simulink model "gru_quadcl"  (Simulink 8.3)
settings: Solver=FixedStepDiscrete  SolverMode=SingleTasking  StartTime=0.0  StopTime=10  FixedStep=0.01  RelTol=1e-3
undefined symbols (not defined in the file): DiscIntNeverNeededParam
libraries: controllibrary x11, simulink x8, snap2lib x3, simulink_need_slupdate x3, utilitylib x2
settings Model: Creator=simon  LastModifiedBy=Robin
settings DataIOCC: LimitDataPoints=off  SaveOutput=off  SignalLogging=off  SaveTime=off
settings OptimizationCC: InlineParams=on  InlineInvariantSignals=on  ExpressionDepthLimit=2147483647  InitFltsAndDblsToZero=on  OptimizeModelRefInitCode=on  LifeSpan=1
settings DebuggingCC: SaveWithParameterizedLinksMsg=none  SignalResolutionControl=TryResolveAllWithWarning  MultiTaskDSMMsg=warning  MultiTaskCondExecSysMsg=none  FcnCallInpInsideContextMsg=UseLocalSettings
settings HardwareCC: TargetLongLongMode=on  TargetIntDivRoundTo=Zero  TargetEndianess=LittleEndian  TargetHWDeviceType=MATLAB Host  ProdEqTarget=off
settings ModelReferenceCC: ModelReferenceNumInstancesAllowed=Single
settings SFSimCC: SimParseCustomCode=off
settings RTWCC: SystemTargetFile=ert_shrlib.tlc  GenCodeOnly=on  TemplateMakefile=ert_default_tmf  PostCodeGenCommand=packNGo(buildInfo, {'packType' 'hierarchical'})  Description=Embedded Coder (host-based shared library target)  ProcessScript=ert_shrlib_make_rtw_hook  IncludeERTFirstTime=on
settings CodeAppCC: IgnoreCustomStorageClasses=off
settings STFCustomTargetCC: GenerateSampleERTMain=on  ParMdlRefBuildCompliant=on  CompOptLevelCompliant=on  CombineOutputUpdateFcns=on  ERTCustomFileBanners=on  SupportContinuousTime=off  SupportNonInlinedSFcns=off  MATLABClassNameForMDSCustomization=Simulink.SoftwareTarget.ERTCustomization  ModelStepFunctionPrototypeControlCompliant=on  GRTInterface=off  SystemTargetFile=ert_shrlib.tlc
settings ERTTargetCC: MultiwordLength=2048  GenerateSampleERTMain=on  ConcurrentExecutionCompliant=off  ERTFirstTimeCompliant=off  CPPClassGenCompliant=off  InlinedParameterPlacement=NonHierarchical  ERTCustomFileTemplate=example_file_process.tlc  ConvertIfToSwitch=off  SuppressUnreachableDefaultCases=off

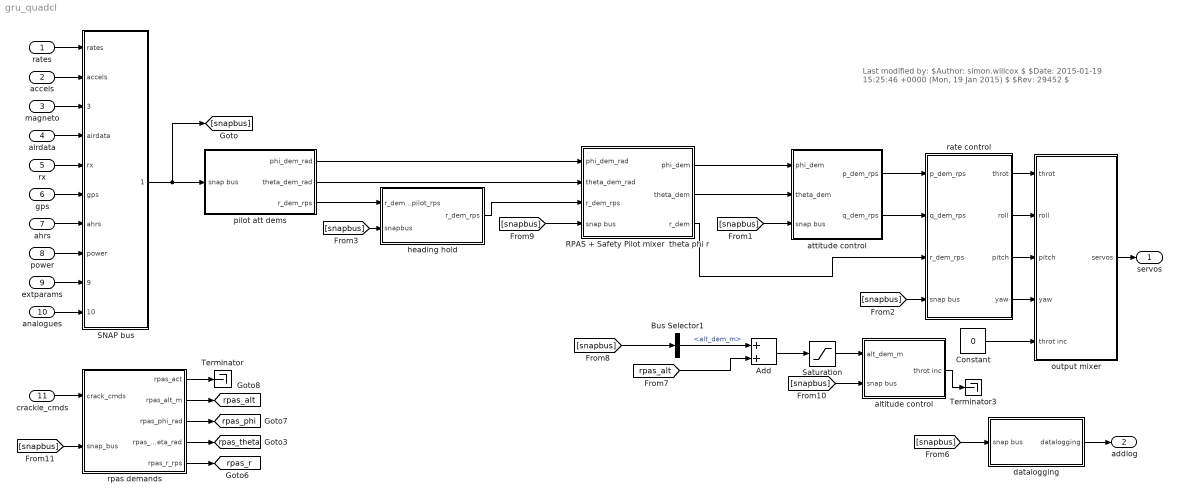
== system gru_quadcl ==
  note: Last modified by:
      | $Author: simon.willcox $
      | $Date: 2015-01-19 15:25:46 +0000 (Mon, 19 Jan 2015) $
      | $Rev: 29452 $
  rates : Inport  PortDimensions=3  SampleTime=0.01
  accels : Inport  Port=2  PortDimensions=3  SampleTime=0.01
  magneto : Inport  Port=3  PortDimensions=3  SampleTime=0.01
  airdata : Inport  Port=4  PortDimensions=3  SampleTime=0.01
  rx : Inport  Port=5  PortDimensions=8  SampleTime=0.01
  gps : Inport  Port=6  PortDimensions=9  SampleTime=0.01
  ahrs : Inport  Port=7  PortDimensions=4  SampleTime=0.01
  power : Inport  Port=8  PortDimensions=3  SampleTime=0.01
  extparams : Inport  Port=9  PortDimensions=64  SampleTime=0.01
  analogues : Inport  Port=10  PortDimensions=8  SampleTime=0.01
  crackle_cmds : Inport  Port=11  PortDimensions=32  SampleTime=0.01
  Add : Sum
  Bus Selector1 : BusSelector  OutputSignals=extbus.alt_dem_m
  Constant : Constant  Value=0
  RPAS + Safety Pilot mixer  theta phi r : Subsystem
  SNAP bus : Subsystem
  Saturation : Saturate  UpperLimit=5  LowerLimit=0
  Terminator : Terminator
  Terminator3 : Terminator
  altitude control : Subsystem
  attitude control : Subsystem
  datalogging : Subsystem  AncestorBlock=snap2lib/datalogging
  heading hold : Subsystem
  output mixer : Subsystem
  pilot att dems : Subsystem
  rate control : Subsystem
  rpas demands : Subsystem
  servos : Outport  PortDimensions=8
  addlog : Outport  Port=2  PortDimensions=32
  tag scope: rpas_alt=global, rpas_phi=global, rpas_r=global, rpas_theta=global
  wires:
  rates/1 -> SNAP bus/1(rates)
  accels/1 -> SNAP bus/2(accels)
  airdata/1 -> SNAP bus/4(airdata)
  power/1 -> SNAP bus/8(power)
  rx/1 -> SNAP bus/5(rx)
  gps/1 -> SNAP bus/6(gps)
  datalogging/1(datalogging) -> addlog/1
  ahrs/1 -> SNAP bus/7(ahrs)
  extparams/1 -> SNAP bus/9(extparams)
  output mixer/1(servos) -> servos/1
  magneto/1 -> SNAP bus/3(magneto)
  analogues/1 -> SNAP bus/10(analogues)
  rate control/1(throt) -> output mixer/1(throt)
  rate control/2(roll) -> output mixer/2(roll)
  [snapbus] -> datalogging/1(snap bus)
  rate control/4(yaw) -> output mixer/4(yaw)
  rate control/3(pitch) -> output mixer/3(pitch)
  SNAP bus/1(snap bus) -> [snapbus], pilot att dems/1(snap bus)
  [snapbus] -> attitude control/3(snap bus)
  [snapbus] -> rate control/4(snap bus)
  Saturation/1 -> altitude control/1(alt_dem_m)
  [snapbus] -> Bus Selector1/1
  rpas demands/1(rpas_act) -> Terminator/1
  rpas demands/2(rpas_alt_m) -> [rpas_alt]
  rpas demands/5(rpas_r_rps) -> [rpas_r]
  rpas demands/3(rpas_phi_rad) -> [rpas_phi]
  rpas demands/4(rpas_theta_rad) -> [rpas_theta]
  [snapbus] -> rpas demands/2(snap_bus)
  crackle_cmds/1 -> rpas demands/1(crack_cmds)
  pilot att dems/1(phi_dem_rad) -> RPAS + Safety Pilot mixer  theta phi r/1(phi_dem_rad)
  RPAS + Safety Pilot mixer  theta phi r/1(phi_dem) -> attitude control/1(phi_dem)
  pilot att dems/2(theta_dem_rad) -> RPAS + Safety Pilot mixer  theta phi r/2(theta_dem_rad)
  RPAS + Safety Pilot mixer  theta phi r/2(theta_dem) -> attitude control/2(theta_dem)
  RPAS + Safety Pilot mixer  theta phi r/3(r_dem) -> rate control/3(r_dem_rps)
  [snapbus] -> RPAS + Safety Pilot mixer  theta phi r/4(snap bus)
  Bus Selector1/1 -> Add/1  "<alt_dem_m>"
  [rpas_alt] -> Add/2
  Add/1 -> Saturation/1
  [snapbus] -> altitude control/2(snap bus)
  altitude control/1(throt inc) -> Terminator3/1
  attitude control/1(p_dem_rps) -> rate control/1(p_dem_rps)
  attitude control/2(q_dem_rps) -> rate control/2(q_dem_rps)
  Constant/1 -> output mixer/5(throt inc)
  [snapbus] -> heading hold/2(snapbus)
  pilot att dems/3(r_dem_rps) -> heading hold/1(r_dem_pilot_rps)
  heading hold/1(r_dem_rps) -> RPAS + Safety Pilot mixer  theta phi r/3(r_dem_rps)

== system gru_quadcl/RPAS + Safety Pilot mixer  theta phi r ==
  phi_dem_rad : Inport
  theta_dem_rad : Inport  Port=2
  r_dem_rps : Inport  Port=3
  snap bus : Inport  Port=4
  Add : Sum
  Add1 : Sum
  Bus Selector5 : BusSelector  OutputSignals=rx.snapact
  Switch3 : Switch  Threshold=0.5
  Switch4 : Switch  Threshold=0.5
  phi_dem : Outport
  theta_dem : Outport  Port=2
  r_dem : Outport  Port=3
  wires:
  phi_dem_rad/1 -> Switch4/3, Add/2
  theta_dem_rad/1 -> Switch3/3, Add1/2
  Add/1 -> Switch4/1
  Add1/1 -> Switch3/1
  Switch4/1 -> phi_dem/1
  Switch3/1 -> theta_dem/1
  r_dem_rps/1 -> r_dem/1
  [rpas_phi] -> Add/1
  [rpas_theta] -> Add1/1
  snap bus/1 -> Bus Selector5/1
  Bus Selector5/1 -> Switch3/2, Switch4/2  "<snapact>"

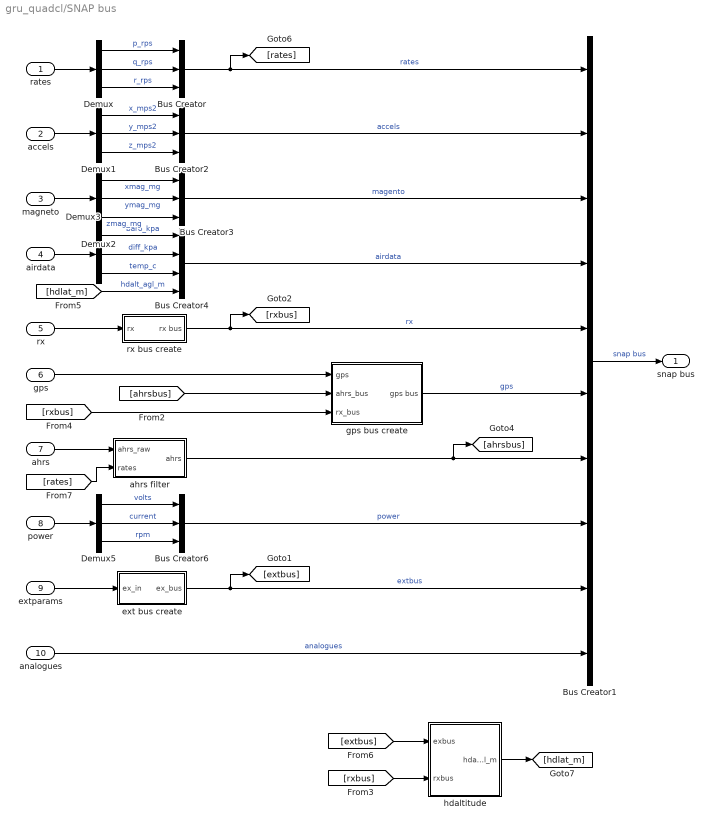
== system gru_quadcl/SNAP bus ==
  rates : Inport  PortDimensions=3
  accels : Inport  Port=2  PortDimensions=3
  magneto : Inport  Port=3  PortDimensions=3
  airdata : Inport  Port=4  PortDimensions=3
  rx : Inport  Port=5  PortDimensions=8
  gps : Inport  Port=6  PortDimensions=9
  ahrs : Inport  Port=7  PortDimensions=4
  power : Inport  Port=8  PortDimensions=3
  extparams : Inport  Port=9  PortDimensions=64
  analogues : Inport  Port=10  PortDimensions=8
  Bus Creator{,2..3,6} (4 alike) : BusCreator  Inputs=3
  Bus Creator1 : BusCreator  Inputs=10
  Bus Creator4 : BusCreator
  Demux{,1..3,5} (5 alike) : Demux  Outputs=3
  ahrs filter : Subsystem
  ext bus create : Subsystem
  gps bus create : Subsystem
  hdaltitude : Subsystem
  rx bus create : Subsystem
  snap bus : Outport
  wires:
  Bus Creator1/1 -> snap bus/1  "snap bus"
  Bus Creator6/1 -> Bus Creator1/8  "power"
  power/1 -> Demux5/1
  Demux5/1 -> Bus Creator6/1  "volts"
  Demux5/2 -> Bus Creator6/2  "current"
  Demux5/3 -> Bus Creator6/3  "rpm"
  ahrs filter/1(ahrs) -> Bus Creator1/7, [ahrsbus]
  ahrs/1 -> ahrs filter/1(ahrs_raw)
  gps bus create/1(gps bus) -> Bus Creator1/6  "gps"
  gps/1 -> gps bus create/1(gps)
  rx bus create/1(rx bus) -> Bus Creator1/5, [rxbus]  "rx"
  Bus Creator4/1 -> Bus Creator1/4  "airdata"
  airdata/1 -> Demux3/1
  Demux3/1 -> Bus Creator4/1  "baro_kpa"
  Demux3/2 -> Bus Creator4/2  "diff_kpa"
  Demux3/3 -> Bus Creator4/3  "temp_c"
  Bus Creator3/1 -> Bus Creator1/3  "magento"
  magneto/1 -> Demux2/1
  Demux2/1 -> Bus Creator3/1  "xmag_mg"
  Demux2/2 -> Bus Creator3/2  "ymag_mg"
  Demux2/3 -> Bus Creator3/3  "zmag_mg"
  Bus Creator2/1 -> Bus Creator1/2  "accels"
  accels/1 -> Demux1/1
  Demux1/1 -> Bus Creator2/1  "x_mps2"
  Demux1/2 -> Bus Creator2/2  "y_mps2"
  Demux1/3 -> Bus Creator2/3  "z_mps2"
  rx/1 -> rx bus create/1(rx)
  rates/1 -> Demux/1
  Bus Creator/1 -> Bus Creator1/1, [rates]  "rates"
  Demux/1 -> Bus Creator/1  "p_rps"
  Demux/2 -> Bus Creator/2  "q_rps"
  Demux/3 -> Bus Creator/3  "r_rps"
  extparams/1 -> ext bus create/1(ex_in)
  ext bus create/1(ex_bus) -> Bus Creator1/9, [extbus]  "extbus"
  analogues/1 -> Bus Creator1/10  "analogues"
  [rxbus] -> gps bus create/3(rx_bus)
  [ahrsbus] -> gps bus create/2(ahrs_bus)
  [rxbus] -> hdaltitude/2(rxbus)
  [extbus] -> hdaltitude/1(exbus)
  [rates] -> ahrs filter/2(rates)
  hdaltitude/1(hdalt_agl_m) -> [hdlat_m]
  [hdlat_m] -> Bus Creator4/4  "hdalt_agl_m"

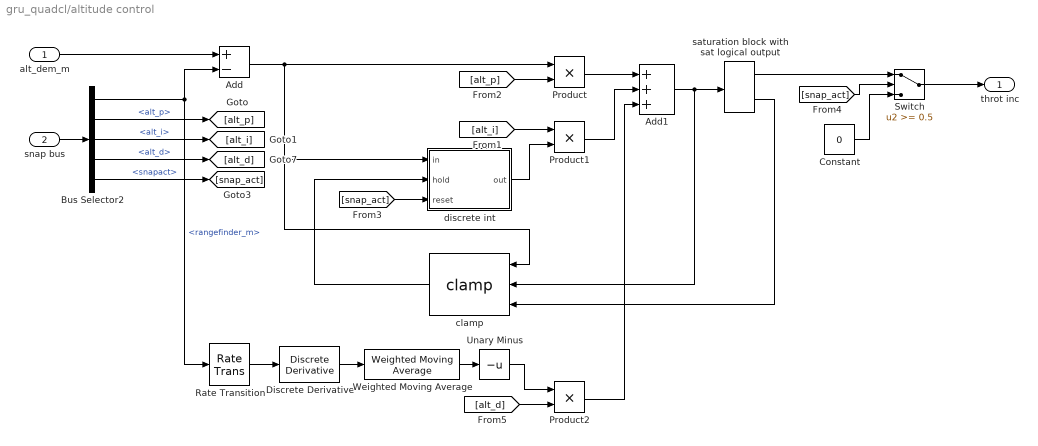
== system gru_quadcl/altitude control ==
  alt_dem_m : Inport
  snap bus : Inport  Port=2
  Add : Sum  Inputs=+-
  Add1 : Sum  Inputs=+++
  Bus Selector2 : BusSelector  OutputSignals=extbus.rangefinder_m,extbus.alt_p,extbus.alt_i,extbus.alt_d,rx.snapact
  Constant : Constant  Value=0
  Discrete Derivative : simulink/Discrete/Discrete Derivative  gainval=1.0  ICPrevScaledInput=0.0  InputProcessing=Inherited  OutMin=[]  OutMax=[]  OutDataType=sfix(16)  OutScaling=2^-10  DoSatur=off
  Product : Product  RndMeth=Zero
  Product1 : Product  RndMeth=Zero
  Product2 : Product  RndMeth=Zero
  Rate Transition : RateTransition  OutPortSampleTime=0.1
  Switch : Switch  Threshold=0.5
  Unary Minus : UnaryMinus
  Weighted Moving Average : simulink_need_slupdate/Weighted Moving Average  mgainval=[0.1 0.1 0.1 0.1 0.1 0.1 0.1 0.1 0.1 0.1]  vinit=0.0  samptime=-1  OutDataType=sfix(16)  OutScaling=2^-10  DoSatur=off  GainDataType=sfix( 16 )  MatRadixGroup=Best Precision: Matrix-wise  GainScaling=2^-10
  clamp : controllibrary/clamp
  discrete int : Subsystem
  saturation block with sat logical output : controllibrary/saturation block with sat logical output  ulim=0.4  llim=-0.25
  throt inc : Outport
  wires:
  [snap_act] -> Switch/2
  Constant/1 -> Switch/3
  Switch/1 -> throt inc/1
  saturation block with sat logical output/1 -> Switch/1
  Bus Selector2/4 -> [alt_d]  "<alt_d>"
  Bus Selector2/5 -> [snap_act]  "<snapact>"
  Bus Selector2/3 -> [alt_i]  "<alt_i>"
  Bus Selector2/2 -> [alt_p]  "<alt_p>"
  saturation block with sat logical output/2 -> clamp/3
  [snap_act] -> discrete int/3(reset)
  [alt_i] -> Product1/1
  [alt_p] -> Product/2
  clamp/1 -> discrete int/2(hold)
  Product1/1 -> Add1/2
  discrete int/1(out) -> Product1/2
  Add1/1 -> clamp/2, saturation block with sat logical output/1
  Product/1 -> Add1/1
  Bus Selector2/1 -> Add/2, Rate Transition/1  "<rangefinder_m>"
  Add/1 -> clamp/1, discrete int/1(in), Product/1
  snap bus/1 -> Bus Selector2/1
  alt_dem_m/1 -> Add/1
  Product2/1 -> Add1/3
  [alt_d] -> Product2/2
  Discrete Derivative/1 -> Weighted Moving Average/1
  Weighted Moving Average/1 -> Unary Minus/1
  Unary Minus/1 -> Product2/1
  Rate Transition/1 -> Discrete Derivative/1

== system gru_quadcl/attitude control ==
  phi_dem : Inport
  theta_dem : Inport  Port=2
  snap bus : Inport  Port=3
  pitch att : Subsystem
  roll att : Subsystem
  snap bus1 : InportShadow  Port=3
  p_dem_rps : Outport
  q_dem_rps : Outport  Port=2
  wires:
  snap bus/1 -> roll att/2(snap bus)
  roll att/1(p_dem_rps) -> p_dem_rps/1
  pitch att/1(q_dem_rps) -> q_dem_rps/1
  snap bus1/1 -> pitch att/2(snap bus)
  phi_dem/1 -> roll att/1(phi_dem_rad)
  theta_dem/1 -> pitch att/1(theta_dem_rad)

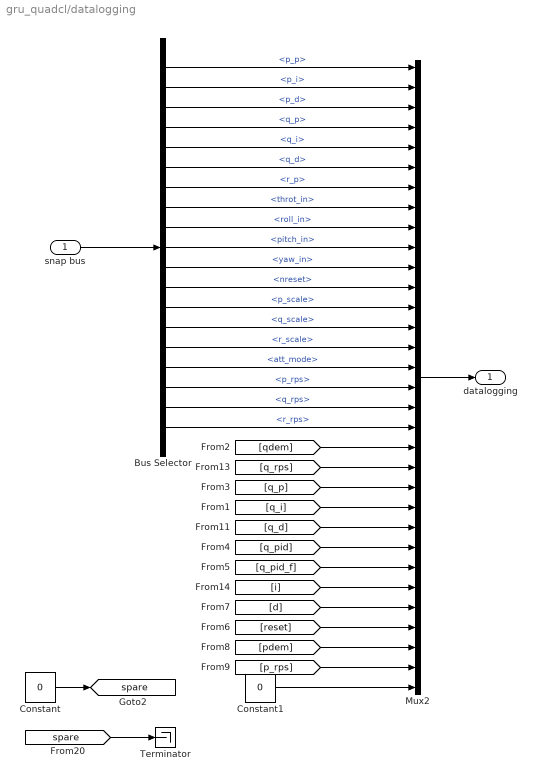
== system gru_quadcl/datalogging ==
  snap bus : Inport
  Bus Selector : BusSelector  OutputSignals=extbus.p_p,extbus.p_i,extbus.p_d,extbus.q_p,extbus.q_i,extbus.q_d,extbus.r_p,rx.throt_in,rx.roll_in,rx.pitch_in,rx.yaw_in,rx.nreset,extbus.p_scale,extbus.q_scale,extbus.r_scale,extbus.att_mode,rates.p_rps,rates.q_rps,rates.r_rps
  Constant : Constant  Value=0
  Constant1 : Constant  Value=0
  Mux2 : Mux  Inputs=32
  Terminator : Terminator
  datalogging : Outport
  tag scope: spare=global
  wires:
  Mux2/1 -> datalogging/1
  Constant/1 -> [spare]
  [spare] -> Terminator/1
  snap bus/1 -> Bus Selector/1
  Bus Selector/1 -> Mux2/1  "<p_p>"
  Bus Selector/3 -> Mux2/3  "<p_d>"
  Bus Selector/2 -> Mux2/2  "<p_i>"
  Bus Selector/7 -> Mux2/7  "<r_p>"
  Bus Selector/8 -> Mux2/8  "<throt_in>"
  Bus Selector/13 -> Mux2/13  "<p_scale>"
  Bus Selector/14 -> Mux2/14  "<q_scale>"
  Bus Selector/11 -> Mux2/11  "<yaw_in>"
  Bus Selector/12 -> Mux2/12  "<nreset>"
  Bus Selector/10 -> Mux2/10  "<pitch_in>"
  Bus Selector/9 -> Mux2/9  "<roll_in>"
  Bus Selector/15 -> Mux2/15  "<r_scale>"
  Bus Selector/4 -> Mux2/4  "<q_p>"
  Bus Selector/6 -> Mux2/6  "<q_d>"
  Bus Selector/5 -> Mux2/5  "<q_i>"
  Bus Selector/16 -> Mux2/16  "<att_mode>"
  Bus Selector/17 -> Mux2/17  "<p_rps>"
  Bus Selector/18 -> Mux2/18  "<q_rps>"
  Bus Selector/19 -> Mux2/19  "<r_rps>"
  [q_pid] -> Mux2/25
  [q_d] -> Mux2/24
  Constant1/1 -> Mux2/32
  [pdem] -> Mux2/30
  [p_rps] -> Mux2/31
  [reset] -> Mux2/29
  [d] -> Mux2/28
  [q_pid_f] -> Mux2/26
  [i] -> Mux2/27
  [q_i] -> Mux2/23
  [q_p] -> Mux2/22
  [q_rps] -> Mux2/21
  [qdem] -> Mux2/20

== system gru_quadcl/heading hold ==
  r_dem_pilot_rps : Inport
  snapbus : Inport  Port=2
  Abs : Abs
  Bus Selector6 : BusSelector  OutputSignals=extbus.r_breakout,ahrs.psi_rad,extbus.head_p
  Dead Zone Dynamic : simulink/Discontinuities/Dead Zone Dynamic
  Product : Product  RndMeth=Zero
  Relational Operator : RelationalOperator  Operator=<  OutDataTypeStr=boolean
  Switch : Switch  Threshold=0.5
  Terminator : Terminator
  Unary Minus : UnaryMinus
  grab heading : Subsystem  TreatAsAtomicUnit=on
  heading error Condition to +/-pi : snap2lib/heading error Condition to +//-pi
  r_dem_pilot_rps1 : InportShadow
  saturation block with sat logical output : controllibrary/saturation block with sat logical output  ulim=30*pi/180  llim=-30*pi/180
  r_dem_rps : Outport
  wires:
  snapbus/1 -> Bus Selector6/1
  Abs/1 -> Relational Operator/1
  Bus Selector6/1 -> Relational Operator/2, [rbreak]  "<r_breakout>"
  Relational Operator/1 -> grab heading/Trigger, Switch/2
  r_dem_pilot_rps/1 -> Abs/1
  grab heading/1(out) -> heading error Condition to +/-pi/1
  heading error Condition to +/-pi/1 -> Product/1
  Bus Selector6/2 -> grab heading/1(in), heading error Condition to +/-pi/2  "<psi_rad>"
  Product/1 -> saturation block with sat logical output/1
  saturation block with sat logical output/2 -> Terminator/1
  saturation block with sat logical output/1 -> Switch/1
  Dead Zone Dynamic/1 -> Switch/3
  Switch/1 -> r_dem_rps/1
  Bus Selector6/3 -> Product/2  "<head_p>"
  r_dem_pilot_rps1/1 -> Dead Zone Dynamic/2
  Unary Minus/1 -> Dead Zone Dynamic/3
  [rbreak] -> Dead Zone Dynamic/1, Unary Minus/1

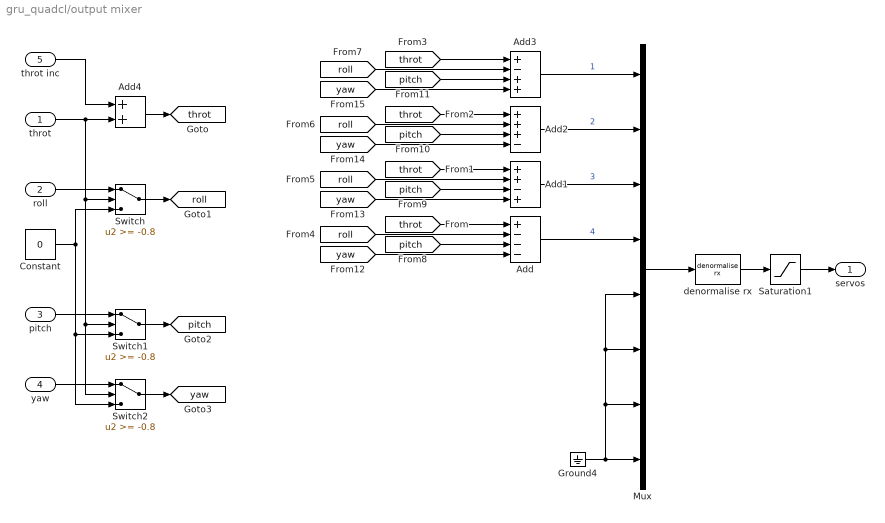
== system gru_quadcl/output mixer ==
  throt : Inport
  roll : Inport  Port=2
  pitch : Inport  Port=3
  yaw : Inport  Port=4
  throt inc : Inport  Port=5
  Add : Sum  Inputs=+---
  Add1 : Sum  Inputs=++-+
  Add2 : Sum  Inputs=+++-
  Add3 : Sum  Inputs=+-++
  Add4 : Sum
  Constant : Constant  Value=0
  Ground4 : Ground
  Mux : Mux  Inputs=8
  Saturation1 : Saturate  UpperLimit=20000  LowerLimit=9000
  Switch : Switch  Threshold=-0.8
  Switch1 : Switch  Threshold=-0.8
  Switch2 : Switch  Threshold=-0.8
  denormalise rx : snap2lib/denormalise rx
  servos : Outport
  tag scope: pitch=global, roll=global, throt=global, yaw=global
  wires:
  Mux/1 -> denormalise rx/1
  denormalise rx/1 -> Saturation1/1
  throt/1 -> Switch/2, Switch1/2, Switch2/2, Add4/2
  Ground4/1 -> Mux/8, Mux/5, Mux/6, Mux/7
  [throt] -> Add/1
  [throt] -> Add1/1
  [throt] -> Add2/1
  [throt] -> Add3/1
  [roll] -> Add/2
  [roll] -> Add1/2
  [roll] -> Add2/2
  [roll] -> Add3/2
  [pitch] -> Add/3
  [pitch] -> Add1/3
  [pitch] -> Add2/3
  [pitch] -> Add3/3
  [yaw] -> Add/4
  [yaw] -> Add1/4
  [yaw] -> Add2/4
  [yaw] -> Add3/4
  roll/1 -> Switch/1
  Switch/1 -> [roll]
  Constant/1 -> Switch/3, Switch1/3, Switch2/3
  pitch/1 -> Switch1/1
  Switch1/1 -> [pitch]
  yaw/1 -> Switch2/1
  Switch2/1 -> [yaw]
  Add4/1 -> [throt]
  throt inc/1 -> Add4/1
  Add/1 -> Mux/4  "4"
  Add1/1 -> Mux/3  "3"
  Add2/1 -> Mux/2  "2"
  Add3/1 -> Mux/1  "1"
  Saturation1/1 -> servos/1

== system gru_quadcl/pilot att dems ==
  snap bus : Inport
  Bus Selector : BusSelector  OutputSignals=rx.roll_in,extbus.phi_scale
  Bus Selector1 : BusSelector  OutputSignals=rx.pitch_in,extbus.theta_scale
  Bus Selector2 : BusSelector  OutputSignals=rx.yaw_in,extbus.r_scale
  Product1 : Product  RndMeth=Zero
  Product2 : Product  RndMeth=Zero
  Product3 : Product  RndMeth=Zero
  p dem scale : Gain  Gain=pi/180
  p dem scale1 : Gain  Gain=pi/180
  p dem scale2 : Gain  Gain=pi/180
  phi_dem_rad : Outport
  theta_dem_rad : Outport  Port=2
  r_dem_rps : Outport  Port=3
  wires:
  Bus Selector/2 -> Product1/2  "<phi_scale>"
  Bus Selector/1 -> Product1/1  "<roll_in>"
  Product1/1 -> p dem scale/1
  Bus Selector1/2 -> Product2/2  "<theta_scale>"
  Bus Selector1/1 -> Product2/1  "<pitch_in>"
  Product2/1 -> p dem scale1/1
  p dem scale/1 -> phi_dem_rad/1
  p dem scale1/1 -> theta_dem_rad/1
  snap bus/1 -> Bus Selector/1, Bus Selector1/1, Bus Selector2/1
  p dem scale2/1 -> r_dem_rps/1
  Product3/1 -> p dem scale2/1
  Bus Selector2/1 -> Product3/1  "<yaw_in>"
  Bus Selector2/2 -> Product3/2  "<r_scale>"

== system gru_quadcl/rate control ==
  p_dem_rps : Inport
  q_dem_rps : Inport  Port=2
  r_dem_rps : Inport  Port=3
  snap bus : Inport  Port=4
  Bus Selector1 : BusSelector  OutputSignals=rx.throt_in
  pitch rate : Subsystem
  roll rate : Subsystem
  snap bus1 : InportShadow  Port=4
  snap bus2 : InportShadow  Port=4
  snap bus3 : InportShadow  Port=4
  yaw rate : Subsystem
  throt : Outport
  roll : Outport  Port=2
  pitch : Outport  Port=3
  yaw : Outport  Port=4
  tag scope: pitchsat=global, rollsat=global
  wires:
  pitch rate/2(sat) -> [pitchsat]
  pitch rate/1(pitch) -> pitch/1
  snap bus1/1 -> pitch rate/2(snap bus)
  q_dem_rps/1 -> pitch rate/1(q_dem_rps)
  roll rate/2(sat) -> [rollsat]
  r_dem_rps/1 -> yaw rate/1(r_dem_rps)
  p_dem_rps/1 -> roll rate/1(p_dem_rps)
  snap bus3/1 -> Bus Selector1/1
  snap bus2/1 -> yaw rate/2(snap bus)
  yaw rate/1(yaw) -> yaw/1
  roll rate/1(roll) -> roll/1
  Bus Selector1/1 -> throt/1  "<throt_in>"
  snap bus/1 -> roll rate/2(snap bus)

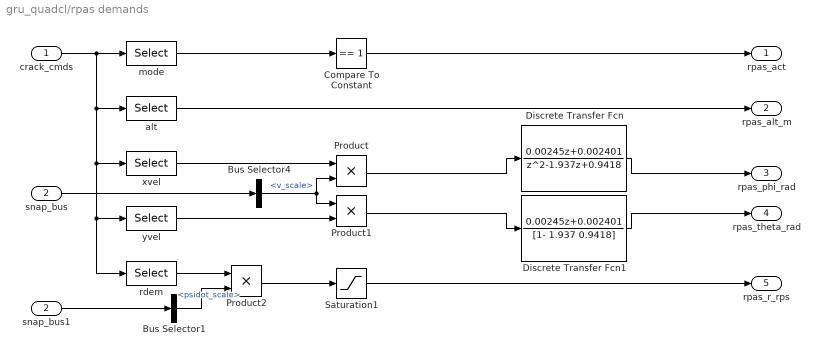
== system gru_quadcl/rpas demands ==
  crack_cmds : Inport
  snap_bus : Inport  Port=2
  Bus Selector1 : BusSelector  OutputSignals=extbus.psidot_scale
  Bus Selector4 : BusSelector  OutputSignals=extbus.v_scale
  Compare To Constant : simulink/Logic and Bit Operations/Compare To Constant  relop===  const=1  OutDataTypeStr=boolean
  Discrete Transfer Fcn : DiscreteTransferFcn  Numerator=[0.00245 0.002401]  Denominator=[1 -1.937 0.9418]
  Discrete Transfer Fcn1 : DiscreteTransferFcn  Numerator=[0.00245 0.002401]  Denominator=[1- 1.937 0.9418]
  Product : Product  RndMeth=Zero
  Product1 : Product  RndMeth=Zero
  Product2 : Product  RndMeth=Zero
  Saturation1 : Saturate
  alt : Selector  IndexMode=Zero-based  InputPortWidth=32
  mode : Selector  IndexMode=Zero-based  InputPortWidth=32  Indices=0
  rdem : Selector  IndexMode=Zero-based  InputPortWidth=32  Indices=4
  snap_bus1 : InportShadow  Port=2
  xvel : Selector  IndexMode=Zero-based  InputPortWidth=32  Indices=3
  yvel : Selector  IndexMode=Zero-based  InputPortWidth=32  Indices=5
  rpas_act : Outport
  rpas_alt_m : Outport  Port=2
  rpas_phi_rad : Outport  Port=3
  rpas_theta_rad : Outport  Port=4
  rpas_r_rps : Outport  Port=5
  wires:
  Bus Selector1/1 -> Product2/2  "<psidot_scale>"
  Product2/1 -> Saturation1/1
  rdem/1 -> Product2/1
  snap_bus/1 -> Bus Selector4/1
  alt/1 -> rpas_alt_m/1
  Compare To Constant/1 -> rpas_act/1
  Bus Selector4/1 -> Product1/1, Product/2  "<v_scale>"
  yvel/1 -> Product1/2
  xvel/1 -> Product/1
  Saturation1/1 -> rpas_r_rps/1
  mode/1 -> Compare To Constant/1
  crack_cmds/1 -> alt/1, yvel/1, rdem/1, xvel/1, mode/1
  snap_bus1/1 -> Bus Selector1/1
  Product/1 -> Discrete Transfer Fcn/1
  Product1/1 -> Discrete Transfer Fcn1/1
  Discrete Transfer Fcn/1 -> rpas_phi_rad/1
  Discrete Transfer Fcn1/1 -> rpas_theta_rad/1

== system gru_quadcl/SNAP bus/ahrs filter ==
  ahrs_raw : Inport
  rates : Inport  Port=2
  Add2 : Sum
  Add3 : Sum  Inputs=-+
  Add4 : Sum
  Bus Creator5 : BusCreator  Inputs=5
  Bus Selector4 : BusSelector  OutputSignals=r_rps
  Demux4 : Demux
  Gain4 : Gain  Gain=0.02
  Memory1 : Memory
  condition angle to +/-pi : utilitylib/condition angle to +//-pi
  condition angle to +/-pi1 : utilitylib/condition angle to +//-pi
  dt : Gain  Gain=0.01
  ahrs : Outport
  wires:
  Demux4/4 -> Bus Creator5/4, [maghead]  "maghead_rad"
  Demux4/1 -> Bus Creator5/1  "phi_rad"
  Demux4/2 -> Bus Creator5/2  "theta_rad"
  Demux4/3 -> Bus Creator5/3  "psi_rad"
  Bus Creator5/1 -> ahrs/1  "ahrs"
  ahrs_raw/1 -> Demux4/1
  rates/1 -> Bus Selector4/1
  Bus Selector4/1 -> dt/1  "<r_rps>"
  dt/1 -> Add2/1
  [estpsi] -> Memory1/1
  Memory1/1 -> Add2/2, Add3/1
  Add2/1 -> Add4/1
  Gain4/1 -> Add4/2
  Add3/1 -> condition angle to +/-pi/1
  condition angle to +/-pi/1 -> Gain4/1
  Add4/1 -> condition angle to +/-pi1/1, [estpsi]
  condition angle to +/-pi1/1 -> Bus Creator5/5  "estpsi_rad"
  [maghead] -> Add3/2

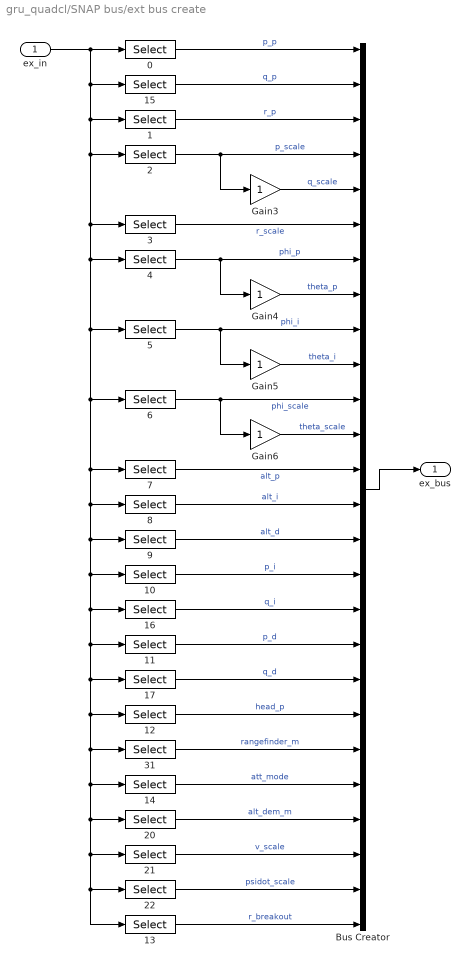
== system gru_quadcl/SNAP bus/ext bus create ==
  ex_in : Inport
  0 : Selector  IndexMode=Zero-based  Indices=0
  1 : Selector  IndexMode=Zero-based
  10 : Selector  IndexMode=Zero-based  Indices=10
  11 : Selector  IndexMode=Zero-based  Indices=11
  12 : Selector  IndexMode=Zero-based  Indices=12
  13 : Selector  IndexMode=Zero-based  Indices=13
  14 : Selector  IndexMode=Zero-based  Indices=14
  15 : Selector  IndexMode=Zero-based  Indices=15
  16 : Selector  IndexMode=Zero-based  Indices=16
  17 : Selector  IndexMode=Zero-based  Indices=17
  2 : Selector  IndexMode=Zero-based  Indices=2
  20 : Selector  IndexMode=Zero-based  Indices=20
  21 : Selector  IndexMode=Zero-based  Indices=21
  22 : Selector  IndexMode=Zero-based  Indices=22
  3 : Selector  IndexMode=Zero-based  Indices=3
  31 : Selector  IndexMode=Zero-based  Indices=31
  4 : Selector  IndexMode=Zero-based  Indices=4
  5 : Selector  IndexMode=Zero-based  Indices=5
  6 : Selector  IndexMode=Zero-based  Indices=6
  7 : Selector  IndexMode=Zero-based  Indices=7
  8 : Selector  IndexMode=Zero-based  Indices=8
  9 : Selector  IndexMode=Zero-based  Indices=9
  Bus Creator : BusCreator  Inputs=26
  Gain{3..6} (4 alike) : Gain
  ex_bus : Outport
  wires:
  Bus Creator/1 -> ex_bus/1
  12/1 -> Bus Creator/20  "head_p"
  9/1 -> Bus Creator/15  "alt_d"
  8/1 -> Bus Creator/14  "alt_i"
  7/1 -> Bus Creator/13  "alt_p"
  Gain6/1 -> Bus Creator/12  "theta_scale"
  Gain5/1 -> Bus Creator/10  "theta_i"
  Gain4/1 -> Bus Creator/8  "theta_p"
  Gain3/1 -> Bus Creator/5  "q_scale"
  15/1 -> Bus Creator/2  "q_p"
  11/1 -> Bus Creator/18  "p_d"
  10/1 -> Bus Creator/16  "p_i"
  6/1 -> Gain6/1, Bus Creator/11  "phi_scale"
  5/1 -> Gain5/1, Bus Creator/9  "phi_i"
  4/1 -> Gain4/1, Bus Creator/7  "phi_p"
  3/1 -> Bus Creator/6  "r_scale"
  2/1 -> Gain3/1, Bus Creator/4  "p_scale"
  1/1 -> Bus Creator/3  "r_p"
  ex_in/1 -> 0/1, 9/1, 10/1, 11/1, 12/1, 31/1, 14/1, 20/1, 21/1, 13/1, 22/1, 17/1, 16/1, 8/1, 7/1, 6/1, 5/1, 4/1, 3/1, 2/1, 1/1, 15/1
  0/1 -> Bus Creator/1  "p_p"
  16/1 -> Bus Creator/17  "q_i"
  31/1 -> Bus Creator/21  "rangefinder_m"
  14/1 -> Bus Creator/22  "att_mode"
  17/1 -> Bus Creator/19  "q_d"
  20/1 -> Bus Creator/23  "alt_dem_m"
  21/1 -> Bus Creator/24  "v_scale"
  22/1 -> Bus Creator/25  "psidot_scale"
  13/1 -> Bus Creator/26  "r_breakout"

== system gru_quadcl/SNAP bus/gps bus create ==
  gps : Inport
  ahrs_bus : Inport  Port=2
  rx_bus : Inport  Port=3
  Bus Creator5 : BusCreator  Inputs=13
  Bus Selector : BusSelector  OutputSignals=nreset
  Bus Selector1 : BusSelector  OutputSignals=estpsi_rad
  Demux4 : Demux  Outputs=9
  RotateVelp : Subsystem
  grab lat/long scaling : Subsystem  AncestorBlock=navlibrary/grab lat//long scaling
  gps bus : Outport
  wires:
  gps/1 -> Demux4/1
  Bus Creator5/1 -> gps bus/1
  Demux4/9 -> Bus Creator5/9  "vdop"
  Demux4/8 -> Bus Creator5/8  "hdop"
  Demux4/7 -> Bus Creator5/7  "pdop"
  Demux4/6 -> Bus Creator5/6  "mode"
  Demux4/5 -> Bus Creator5/5, [head]  "heading_rad"
  Demux4/4 -> Bus Creator5/4, [vel]  "velocity_mps"
  Demux4/3 -> Bus Creator5/3  "altitude_m"
  Demux4/2 -> Bus Creator5/2  "longitude_deg"
  Demux4/1 -> Bus Creator5/1, [latdeg]  "latitude_deg"
  rx_bus/1 -> Bus Selector/1
  Bus Selector/1 -> grab lat/long scaling/Trigger  "<nreset>"
  [latdeg] -> grab lat/long scaling/1(lat_deg)
  [head] -> RotateVelp/1(head_rad)
  [vel] -> RotateVelp/3(vel_mps)
  Bus Selector1/1 -> RotateVelp/2(maghead_rad)  "<estpsi_rad>"
  ahrs_bus/1 -> Bus Selector1/1
  RotateVelp/1(velbx_mps) -> Bus Creator5/10  "velbx_mps"
  RotateVelp/2(velby_mps) -> Bus Creator5/11  "velby_mps"
  grab lat/long scaling/1(long2m) -> Bus Creator5/12  "long2m"
  grab lat/long scaling/2(lat2m) -> Bus Creator5/13  "lat2m"

== system gru_quadcl/SNAP bus/hdaltitude ==
  exbus : Inport
  rxbus : Inport  Port=2
  Add : Sum  Inputs=-+
  Bus Selector3 : BusSelector  OutputSignals=nreset
  Bus Selector4 : BusSelector  OutputSignals=rangefinder_m
  grab alt : Subsystem  TreatAsAtomicUnit=on
  hdalt_agl_m : Outport
  wires:
  exbus/1 -> Bus Selector4/1
  Bus Selector4/1 -> grab alt/1(value), Add/2  "<rangefinder_m>"
  rxbus/1 -> Bus Selector3/1
  Bus Selector3/1 -> grab alt/Trigger  "<nreset>"
  grab alt/1(grabbed value) -> Add/1
  Add/1 -> hdalt_agl_m/1

== system gru_quadcl/SNAP bus/rx bus create ==
  rx : Inport
  Bus Creator5 : BusCreator  Inputs=9
  Compare To Constant : simulink/Logic and Bit Operations/Compare To Constant  relop=>=  const=-0.6  OutDataTypeStr=boolean  ZeroCross=off
  Compare To Zero : simulink/Logic and Bit Operations/Compare To Zero  relop=>=  OutDataTypeStr=boolean  ZeroCross=off
  Compare To Zero1 : simulink/Logic and Bit Operations/Compare To Zero  relop=>=  OutDataTypeStr=boolean  ZeroCross=off
  Constant : Constant  Value=0
  Data Type Conversion1 : DataTypeConversion  OutDataTypeStr=double
  Data Type Conversion2 : DataTypeConversion  OutDataTypeStr=double
  Data Type Conversion3 : DataTypeConversion  OutDataTypeStr=double
  Demux4 : Demux  Outputs=8
  Gain : Gain  Gain=-1
  Logical Operator : Logic  Operator=NOT  AllPortsSameDT=off  OutDataTypeStr=boolean
  Terminator : Terminator
  normalise rx : snap2lib/normalise rx
  rx bus : Outport
  wires:
  normalise rx/1 -> Demux4/1
  rx/1 -> normalise rx/1
  Bus Creator5/1 -> rx bus/1
  Demux4/1 -> Bus Creator5/1, Compare To Constant/1  "throt_in"
  Compare To Zero1/1 -> Data Type Conversion1/1
  Compare To Zero/1 -> Data Type Conversion2/1
  Logical Operator/1 -> Data Type Conversion3/1
  Compare To Constant/1 -> Logical Operator/1
  Data Type Conversion3/1 -> [nreset]
  Demux4/2 -> Terminator/1
  Demux4/3 -> Bus Creator5/2  "roll_in"
  Demux4/4 -> Gain/1  "pitch_in"
  Demux4/5 -> Bus Creator5/4  "yaw_in"
  Demux4/6 -> Compare To Zero/1  "rx6"
  Data Type Conversion2/1 -> Bus Creator5/5  "snapact"
  Demux4/7 -> Compare To Zero1/1  "rx7"
  Data Type Conversion1/1 -> Bus Creator5/6  "hhold"
  Demux4/8 -> Bus Creator5/7  "rx8"
  Constant/1 -> Bus Creator5/8
  [nreset] -> Bus Creator5/9  "nreset"
  Gain/1 -> Bus Creator5/3  "pitch_in"

== system gru_quadcl/altitude control/discrete int ==
  in : Inport
  hold : Inport  Port=2
  reset : Inport  Port=3
  Constant : Constant  Value=0
  Discrete-Time Integrator : DiscreteIntegrator  ExternalReset=rising  SampleTime=0.01  ICPrevOutput=DiscIntNeverNeededParam  ICPrevScaledInput=DiscIntNeverNeededParam
  Switch : Switch  Threshold=0.5
  out : Outport
  wires:
  reset/1 -> Discrete-Time Integrator/2
  in/1 -> Switch/3
  Discrete-Time Integrator/1 -> out/1
  hold/1 -> Switch/2
  Constant/1 -> Switch/1
  Switch/1 -> Discrete-Time Integrator/1

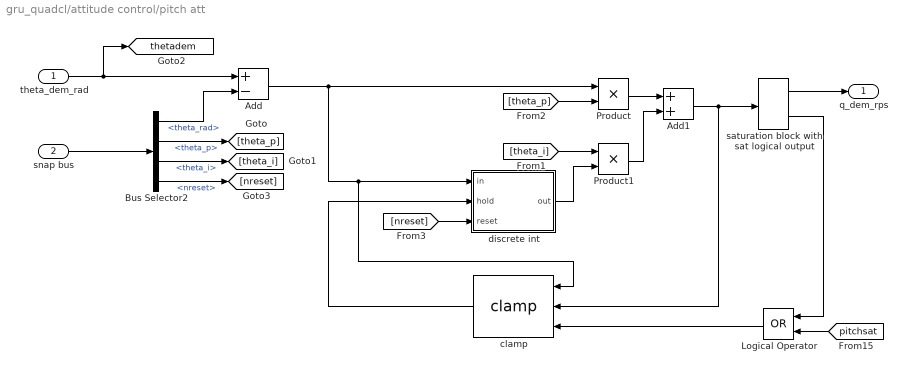
== system gru_quadcl/attitude control/pitch att ==
  theta_dem_rad : Inport
  snap bus : Inport  Port=2
  Add : Sum  Inputs=+-
  Add1 : Sum
  Bus Selector2 : BusSelector  OutputSignals=ahrs.theta_rad,extbus.theta_p,extbus.theta_i,rx.nreset
  Logical Operator : Logic  Operator=OR  AllPortsSameDT=off  OutDataTypeStr=boolean
  Product : Product  RndMeth=Zero
  Product1 : Product  RndMeth=Zero
  clamp : controllibrary/clamp
  discrete int : Subsystem
  saturation block with sat logical output : controllibrary/saturation block with sat logical output  ulim=pi  llim=-pi
  q_dem_rps : Outport
  tag scope: thetadem=global
  wires:
  Logical Operator/1 -> clamp/3
  [pitchsat] -> Logical Operator/2
  saturation block with sat logical output/2 -> Logical Operator/1
  saturation block with sat logical output/1 -> q_dem_rps/1
  theta_dem_rad/1 -> [thetadem], Add/1
  snap bus/1 -> Bus Selector2/1
  Add/1 -> Product/1, discrete int/1(in), clamp/1
  Bus Selector2/1 -> Add/2  "<theta_rad>"
  Product/1 -> Add1/1
  Add1/1 -> saturation block with sat logical output/1, clamp/2
  discrete int/1(out) -> Product1/2
  Product1/1 -> Add1/2
  clamp/1 -> discrete int/2(hold)
  Bus Selector2/2 -> [theta_p]  "<theta_p>"
  Bus Selector2/3 -> [theta_i]  "<theta_i>"
  [theta_p] -> Product/2
  [theta_i] -> Product1/1
  [nreset] -> discrete int/3(reset)
  Bus Selector2/4 -> [nreset]  "<nreset>"

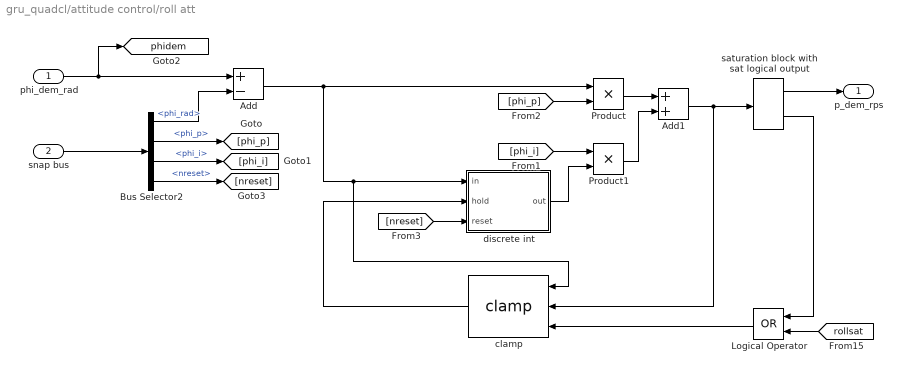
== system gru_quadcl/attitude control/roll att ==
  phi_dem_rad : Inport
  snap bus : Inport  Port=2
  Add : Sum  Inputs=+-
  Add1 : Sum
  Bus Selector2 : BusSelector  OutputSignals=ahrs.phi_rad,extbus.phi_p,extbus.phi_i,rx.nreset
  Logical Operator : Logic  Operator=OR  AllPortsSameDT=off  OutDataTypeStr=boolean
  Product : Product  RndMeth=Zero
  Product1 : Product  RndMeth=Zero
  clamp : controllibrary/clamp
  discrete int : Subsystem
  saturation block with sat logical output : controllibrary/saturation block with sat logical output  ulim=pi  llim=-pi
  p_dem_rps : Outport
  tag scope: phidem=global
  wires:
  [rollsat] -> Logical Operator/2
  saturation block with sat logical output/2 -> Logical Operator/1
  Logical Operator/1 -> clamp/3
  [nreset] -> discrete int/3(reset)
  [phi_i] -> Product1/1
  [phi_p] -> Product/2
  Bus Selector2/3 -> [phi_i]  "<phi_i>"
  Bus Selector2/2 -> [phi_p]  "<phi_p>"
  clamp/1 -> discrete int/2(hold)
  Product1/1 -> Add1/2
  discrete int/1(out) -> Product1/2
  Add1/1 -> clamp/2, saturation block with sat logical output/1
  Product/1 -> Add1/1
  Bus Selector2/1 -> Add/2  "<phi_rad>"
  Add/1 -> clamp/1, discrete int/1(in), Product/1
  snap bus/1 -> Bus Selector2/1
  phi_dem_rad/1 -> Add/1, [phidem]
  saturation block with sat logical output/1 -> p_dem_rps/1
  Bus Selector2/4 -> [nreset]  "<nreset>"

== system gru_quadcl/heading hold/grab heading ==
  in : Inport
  Trigger : TriggerPort
  out : Outport
  wires:
  in/1 -> out/1

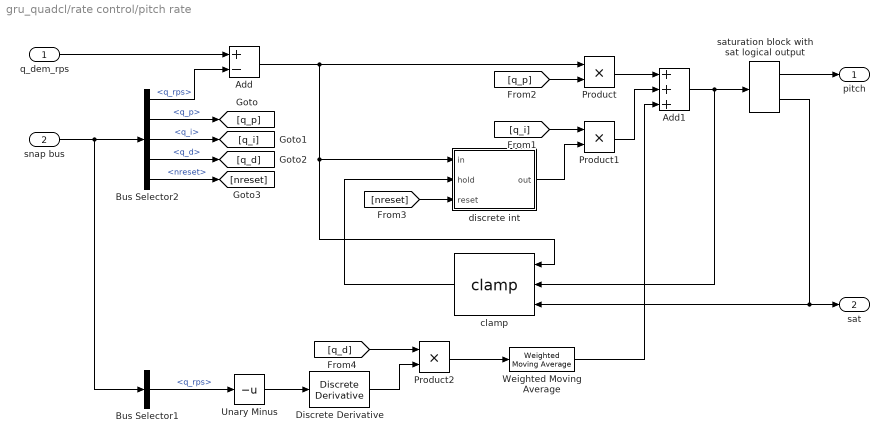
== system gru_quadcl/rate control/pitch rate ==
  q_dem_rps : Inport
  snap bus : Inport  Port=2
  Add : Sum  Inputs=+-
  Add1 : Sum  Inputs=+++
  Bus Selector1 : BusSelector  OutputSignals=rates.q_rps
  Bus Selector2 : BusSelector  OutputSignals=rates.q_rps,extbus.q_p,extbus.q_i,extbus.q_d,rx.nreset
  Discrete Derivative : simulink/Discrete/Discrete Derivative  gainval=1.0  ICPrevScaledInput=0.0  InputProcessing=Inherited  OutMin=[]  OutMax=[]  OutDataType=sfix(16)  OutScaling=2^-10  DoSatur=off
  Product : Product  RndMeth=Zero
  Product1 : Product  RndMeth=Zero
  Product2 : Product  RndMeth=Zero
  Unary Minus : UnaryMinus
  Weighted Moving Average : simulink_need_slupdate/Weighted Moving Average  mgainval=[0.5 0.5]  vinit=0.0  samptime=-1  OutDataType=sfix(16)  OutScaling=2^-10  DoSatur=off  GainDataType=sfix( 16 )  MatRadixGroup=Best Precision: Matrix-wise  GainScaling=2^-10
  clamp : controllibrary/clamp
  discrete int : Subsystem
  saturation block with sat logical output : controllibrary/saturation block with sat logical output  ulim=0.4  llim=-0.4
  pitch : Outport
  sat : Outport  Port=2
  wires:
  Weighted Moving Average/1 -> Add1/3
  Bus Selector1/1 -> Unary Minus/1  "<q_rps>"
  Unary Minus/1 -> Discrete Derivative/1
  saturation block with sat logical output/2 -> clamp/3, sat/1
  [nreset] -> discrete int/3(reset)
  [q_i] -> Product1/1
  [q_p] -> Product/2
  Bus Selector2/3 -> [q_i]  "<q_i>"
  Bus Selector2/2 -> [q_p]  "<q_p>"
  clamp/1 -> discrete int/2(hold)
  Product1/1 -> Add1/2
  discrete int/1(out) -> Product1/2
  Add1/1 -> clamp/2, saturation block with sat logical output/1
  Product/1 -> Add1/1
  Bus Selector2/1 -> Add/2  "<q_rps>"
  Add/1 -> clamp/1, discrete int/1(in), Product/1
  snap bus/1 -> Bus Selector1/1, Bus Selector2/1
  q_dem_rps/1 -> Add/1
  saturation block with sat logical output/1 -> pitch/1
  Bus Selector2/4 -> [q_d]  "<q_d>"
  Discrete Derivative/1 -> Product2/2
  [q_d] -> Product2/1
  Product2/1 -> Weighted Moving Average/1
  Bus Selector2/5 -> [nreset]  "<nreset>"

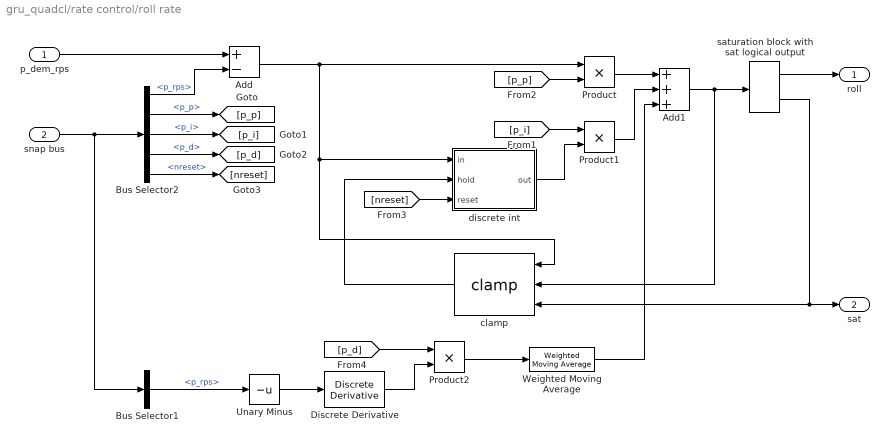
== system gru_quadcl/rate control/roll rate ==
  p_dem_rps : Inport
  snap bus : Inport  Port=2
  Add : Sum  Inputs=+-
  Add1 : Sum  Inputs=+++
  Bus Selector1 : BusSelector  OutputSignals=rates.p_rps
  Bus Selector2 : BusSelector  OutputSignals=rates.p_rps,extbus.p_p,extbus.p_i,extbus.p_d,rx.nreset
  Discrete Derivative : simulink/Discrete/Discrete Derivative  gainval=1.0  ICPrevScaledInput=0.0  InputProcessing=Inherited  OutMin=[]  OutMax=[]  OutDataType=sfix(16)  OutScaling=2^-10  DoSatur=off
  Product : Product  RndMeth=Zero
  Product1 : Product  RndMeth=Zero
  Product2 : Product  RndMeth=Zero
  Unary Minus : UnaryMinus
  Weighted Moving Average : simulink_need_slupdate/Weighted Moving Average  mgainval=[0.5 0.5]  vinit=0.0  samptime=-1  OutDataType=sfix(16)  OutScaling=2^-10  DoSatur=off  GainDataType=sfix( 16 )  MatRadixGroup=Best Precision: Matrix-wise  GainScaling=2^-10
  clamp : controllibrary/clamp
  discrete int : Subsystem
  saturation block with sat logical output : controllibrary/saturation block with sat logical output  ulim=0.2  llim=-0.2
  roll : Outport
  sat : Outport  Port=2
  wires:
  Weighted Moving Average/1 -> Add1/3
  Bus Selector1/1 -> Unary Minus/1  "<p_rps>"
  Unary Minus/1 -> Discrete Derivative/1
  [p_i] -> Product1/1
  Product2/1 -> Weighted Moving Average/1
  [p_d] -> Product2/1
  Discrete Derivative/1 -> Product2/2
  Bus Selector2/4 -> [p_d]  "<p_d>"
  saturation block with sat logical output/1 -> roll/1
  snap bus/1 -> Bus Selector1/1, Bus Selector2/1
  Add/1 -> Product/1, clamp/1, discrete int/1(in)
  Bus Selector2/1 -> Add/2  "<p_rps>"
  Product/1 -> Add1/1
  Add1/1 -> saturation block with sat logical output/1, clamp/2
  discrete int/1(out) -> Product1/2
  Product1/1 -> Add1/2
  clamp/1 -> discrete int/2(hold)
  Bus Selector2/2 -> [p_p]  "<p_p>"
  Bus Selector2/3 -> [p_i]  "<p_i>"
  [p_p] -> Product/2
  [nreset] -> discrete int/3(reset)
  saturation block with sat logical output/2 -> clamp/3, sat/1
  Bus Selector2/5 -> [nreset]  "<nreset>"
  p_dem_rps/1 -> Add/1

== system gru_quadcl/rate control/yaw rate ==
  r_dem_rps : Inport
  snap bus : Inport  Port=2
  Add : Sum  Inputs=+-
  Bus Selector2 : BusSelector  OutputSignals=rates.r_rps,extbus.r_p
  Product : Product  RndMeth=Zero
  Saturation : Saturate  UpperLimit=0.2  LowerLimit=-0.2
  yaw : Outport
  tag scope: rdem=global
  wires:
  Saturation/1 -> yaw/1
  r_dem_rps/1 -> [rdem], Add/1
  Product/1 -> Saturation/1
  snap bus/1 -> Bus Selector2/1
  Bus Selector2/2 -> Product/2  "<r_p>"
  Add/1 -> Product/1
  Bus Selector2/1 -> Add/2  "<r_rps>"

== system gru_quadcl/SNAP bus/gps bus create/RotateVelp ==
  head_rad : Inport
  maghead_rad : Inport  Port=2
  vel_mps : Inport  Port=3
  Product : Product  RndMeth=Zero
  Product1 : Product  RndMeth=Zero
  Subtract : Sum  Inputs=+-
  Trigonometric Function : Trigonometry
  Trigonometric Function1 : Trigonometry  Operator=cos
  velbx_mps : Outport
  velby_mps : Outport  Port=2
  wires:
  head_rad/1 -> Subtract/1
  maghead_rad/1 -> Subtract/2
  Subtract/1 -> Trigonometric Function1/1, Trigonometric Function/1
  Trigonometric Function1/1 -> Product/1
  vel_mps/1 -> Product/2, Product1/1
  Trigonometric Function/1 -> Product1/2
  Product/1 -> velbx_mps/1
  Product1/1 -> velby_mps/1

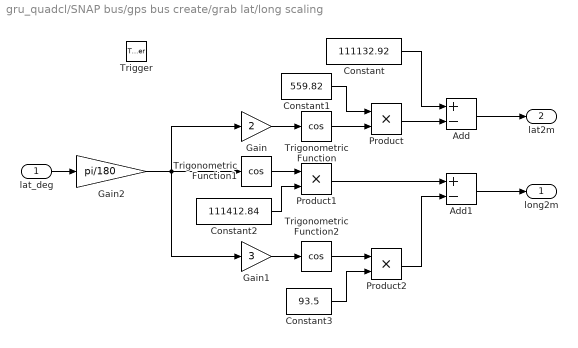
== system gru_quadcl/SNAP bus/gps bus create/grab lat/long scaling ==
  lat_deg : Inport
  Trigger : TriggerPort  TriggerType=falling
  Add : Sum  Inputs=+-
  Add1 : Sum  Inputs=+-
  Constant : Constant  Value=111132.92
  Constant1 : Constant  Value=559.82
  Constant2 : Constant  Value=111412.84
  Constant3 : Constant  Value=93.5
  Gain : Gain  Gain=2
  Gain1 : Gain  Gain=3
  Gain2 : Gain  Gain=pi/180
  Product : Product  RndMeth=Zero
  Product1 : Product  RndMeth=Zero
  Product2 : Product  RndMeth=Zero
  Trigonometric Function : Trigonometry  Operator=cos
  Trigonometric Function1 : Trigonometry  Operator=cos
  Trigonometric Function2 : Trigonometry  Operator=cos
  long2m : Outport  InitialOutput=68481
  lat2m : Outport  Port=2  InitialOutput=111270
  wires:
  Add1/1 -> long2m/1
  Trigonometric Function2/1 -> Product2/1
  Gain1/1 -> Trigonometric Function2/1
  Product1/1 -> Add1/1
  Constant2/1 -> Product1/2
  Trigonometric Function1/1 -> Product1/1
  Add/1 -> lat2m/1
  Product/1 -> Add/2
  Constant1/1 -> Product/1
  Constant/1 -> Add/1
  Trigonometric Function/1 -> Product/2
  Gain/1 -> Trigonometric Function/1
  Gain2/1 -> Gain1/1, Trigonometric Function1/1, Gain/1
  lat_deg/1 -> Gain2/1
  Constant3/1 -> Product2/2
  Product2/1 -> Add1/2

== system gru_quadcl/SNAP bus/hdaltitude/grab alt ==
  value : Inport
  Trigger : TriggerPort  TriggerType=falling
  grabbed value : Outport  InitialOutput=0
  wires:
  value/1 -> grabbed value/1

== system gru_quadcl/attitude control/pitch att/discrete int ==
  in : Inport
  hold : Inport  Port=2
  reset : Inport  Port=3
  Constant : Constant  Value=0
  Discrete-Time Integrator : DiscreteIntegrator  ExternalReset=level  SampleTime=0.01  ICPrevOutput=DiscIntNeverNeededParam  ICPrevScaledInput=DiscIntNeverNeededParam
  Switch : Switch  Threshold=0.5
  out : Outport
  wires:
  Switch/1 -> Discrete-Time Integrator/1
  Constant/1 -> Switch/1
  hold/1 -> Switch/2
  Discrete-Time Integrator/1 -> out/1
  in/1 -> Switch/3
  reset/1 -> Discrete-Time Integrator/2

== system gru_quadcl/attitude control/roll att/discrete int ==
  in : Inport
  hold : Inport  Port=2
  reset : Inport  Port=3
  Constant : Constant  Value=0
  Discrete-Time Integrator : DiscreteIntegrator  ExternalReset=level  SampleTime=0.01  ICPrevOutput=DiscIntNeverNeededParam  ICPrevScaledInput=DiscIntNeverNeededParam
  Switch : Switch  Threshold=0.5
  out : Outport
  wires:
  reset/1 -> Discrete-Time Integrator/2
  in/1 -> Switch/3
  Discrete-Time Integrator/1 -> out/1
  hold/1 -> Switch/2
  Constant/1 -> Switch/1
  Switch/1 -> Discrete-Time Integrator/1

== system gru_quadcl/rate control/pitch rate/discrete int ==
  in : Inport
  hold : Inport  Port=2
  reset : Inport  Port=3
  Constant : Constant  Value=0
  Discrete-Time Integrator : DiscreteIntegrator  ExternalReset=level  SampleTime=0.01  ICPrevOutput=DiscIntNeverNeededParam  ICPrevScaledInput=DiscIntNeverNeededParam
  Switch : Switch  Threshold=0.5
  out : Outport
  wires:
  reset/1 -> Discrete-Time Integrator/2
  in/1 -> Switch/3
  Discrete-Time Integrator/1 -> out/1
  hold/1 -> Switch/2
  Constant/1 -> Switch/1
  Switch/1 -> Discrete-Time Integrator/1

== system gru_quadcl/rate control/roll rate/discrete int ==
  in : Inport
  hold : Inport  Port=2
  reset : Inport  Port=3
  Constant : Constant  Value=0
  Discrete-Time Integrator : DiscreteIntegrator  ExternalReset=level  SampleTime=0.01  ICPrevOutput=DiscIntNeverNeededParam  ICPrevScaledInput=DiscIntNeverNeededParam
  Switch : Switch  Threshold=0.5
  out : Outport
  wires:
  Switch/1 -> Discrete-Time Integrator/1
  Constant/1 -> Switch/1
  hold/1 -> Switch/2
  Discrete-Time Integrator/1 -> out/1
  in/1 -> Switch/3
  reset/1 -> Discrete-Time Integrator/2
